simulink model "untitled22"  (R2019a)
settings: Solver=VariableStepAuto  StartTime=0.0  StopTime=100  RelTol=1e-3
values from neighbouring files (symbols this model uses):
  a0 = 3    [Gradient_instant_cost.m]    (also in Gradient_integral_cost.m; MRAC.m = 3+n(1); MRAC2.m = 1+n(1); MRAC3.m = 1)
  a1 = 2    [Gradient_instant_cost.m]    (also in Gradient_integral_cost.m; MRAC.m = 5+n(2); MRAC2.m = 5+n(2); MRAC3.m = 3)
  am = 1    [Untitled34.m]
  b0 = 1    [Gradient_instant_cost.m]    (also in Gradient_integral_cost.m; MRAC.m = 7+n(3); MRAC2.m = 3+n(3); MRAC3.m = 3)
  lambda = [lambda1; lambda0]    [Gradient_instant_cost.m]    (also in Gradient_integral_cost.m; PureLSQ.m; Untitled2.m = 10; Untitled34.m = 1)
settings Model: Creator=Student  LastModifiedBy=Student

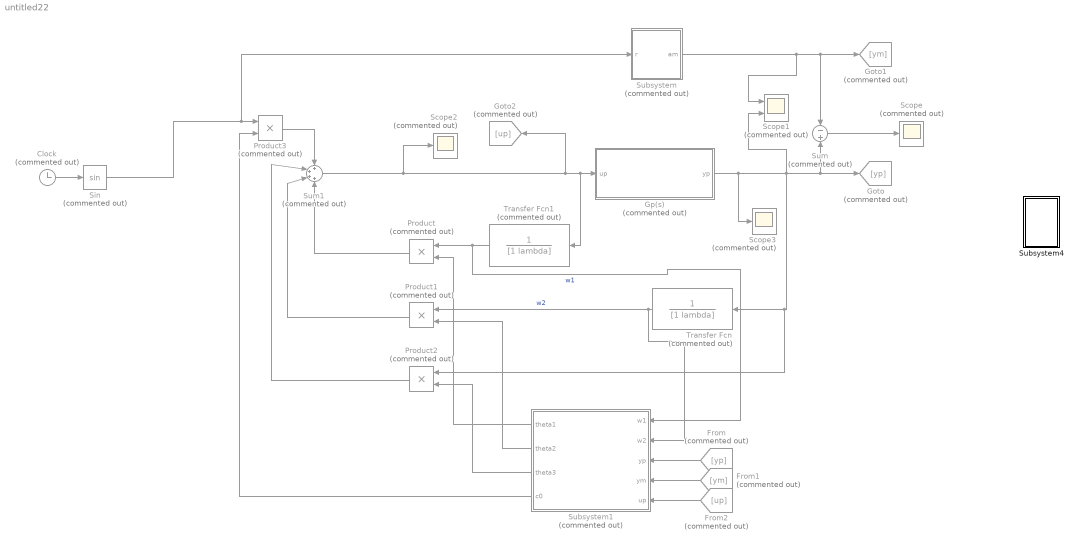
== system untitled22 ==
  Clock : Clock  Commented=on
  From : From  Commented=on  GotoTag=yp
  From1 : From  Commented=on  GotoTag=ym
  From2 : From  Commented=on  GotoTag=up
  Goto : Goto  Commented=on  GotoTag=yp
  Goto1 : Goto  Commented=on  GotoTag=ym
  Goto2 : Goto  Commented=on  GotoTag=up
  Gp(s) : Subsystem  Commented=on
  Product{,1..3} (4 alike) : Product  Commented=on
  Scope : Scope  Commented=on
  Scope1 : Scope  Commented=on  NumInputPorts=2
  Scope2 : Scope  Commented=on
  Scope3 : Scope  Commented=on
  Sin : Trigonometry  Commented=on
  Subsystem : Subsystem  Commented=on
  Subsystem1 : Subsystem  Commented=on
  Subsystem4 : Subsystem
  Sum : Sum  Commented=on  Inputs=-+
  Sum1 : Sum  Commented=on  Inputs=++++
  Transfer Fcn : TransferFcn  Commented=on  Denominator=[1 lambda]
  Transfer Fcn1 : TransferFcn  Commented=on  Denominator=[1 lambda]
  wires:
  Subsystem/1(am) -> Scope1/1, Goto1/1, Sum/1
  Transfer Fcn1/1 -> Subsystem1/1(w1), Product/1  "w1"
  Subsystem1/1(theta1) -> Product/2
  Subsystem1/2(theta2) -> Product1/2
  Transfer Fcn/1 -> Product1/1, Subsystem1/2(w2)  "w2"
  Subsystem1/3(theta3) -> Product2/2
  Product/1 -> Sum1/4
  Product1/1 -> Sum1/3
  Product2/1 -> Sum1/2
  Product3/1 -> Sum1/1
  Subsystem1/4(c0) -> Product3/2
  Gp(s)/1(yp) -> Scope3/1, Product2/1, Transfer Fcn/1, Scope1/2, Goto/1, Sum/2
  From/1 -> Subsystem1/3(yp)
  From1/1 -> Subsystem1/4(ym)
  From2/1 -> Subsystem1/5(up)
  Sum/1 -> Scope/1
  Sin/1 -> Subsystem/1(r), Product3/1
  Sum1/1 -> Scope2/1, Transfer Fcn1/1, Gp(s)/1(up), Goto2/1
  Clock/1 -> Sin/1

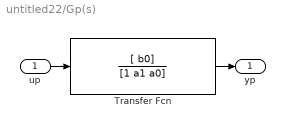
== system untitled22/Gp(s) ==
  up : Inport
  Transfer Fcn : TransferFcn  Numerator=[ b0]  Denominator=[1 a1 a0]
  yp : Outport
  wires:
  Transfer Fcn/1 -> yp/1
  up/1 -> Transfer Fcn/1

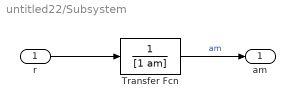
== system untitled22/Subsystem ==
  r : Inport
  Transfer Fcn : TransferFcn  Denominator=[1 am]
  am : Outport
  wires:
  r/1 -> Transfer Fcn/1
  Transfer Fcn/1 -> am/1  "am"

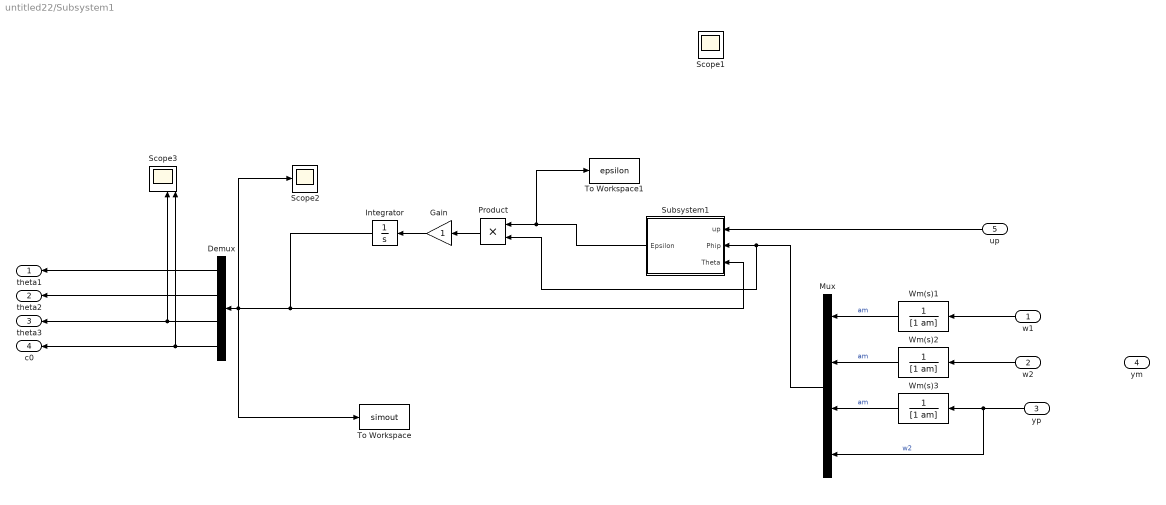
== system untitled22/Subsystem1 ==
  w1 : Inport
  w2 : Inport  Port=2
  yp : Inport  Port=3
  ym : Inport  Port=4
  up : Inport  Port=5
  Demux : Demux
  Gain : Gain
  Integrator : Integrator  InitialCondition=[0;0;0;1]
  Mux : Mux
  Product : Product
  Scope1 : Scope
  Scope2 : Scope
  Scope3 : Scope  NumInputPorts=4
  Subsystem1 : Subsystem
  To Workspace : ToWorkspace  VariableName=simout  SaveFormat=Timeseries  SampleTime=-1
  To Workspace1 : ToWorkspace  VariableName=epsilon  SaveFormat=Timeseries  SampleTime=-1
  Wm(s)1 : TransferFcn  Denominator=[1 am]
  Wm(s)2 : TransferFcn  Denominator=[1 am]
  Wm(s)3 : TransferFcn  Denominator=[1 am]
  theta1 : Outport
  theta2 : Outport  Port=2
  theta3 : Outport  Port=3
  c0 : Outport  Port=4
  wires:
  Demux/3 -> Scope3/3, theta3/1
  Demux/2 -> theta2/1
  Demux/4 -> Scope3/4, c0/1
  Wm(s)1/1 -> Mux/1  "am"
  Wm(s)2/1 -> Mux/2  "am"
  Wm(s)3/1 -> Mux/3  "am"
  Gain/1 -> Integrator/1
  yp/1 -> Mux/4, Wm(s)3/1  "w2"
  Product/1 -> Gain/1
  w1/1 -> Wm(s)1/1
  w2/1 -> Wm(s)2/1
  Demux/1 -> theta1/1
  up/1 -> Subsystem1/1(up)
  Mux/1 -> Product/2, Subsystem1/2(Phip)
  Integrator/1 -> To Workspace/1, Scope2/1, Demux/1, Subsystem1/3(Theta)
  Subsystem1/1("Epsilon ") -> To Workspace1/1, Product/1

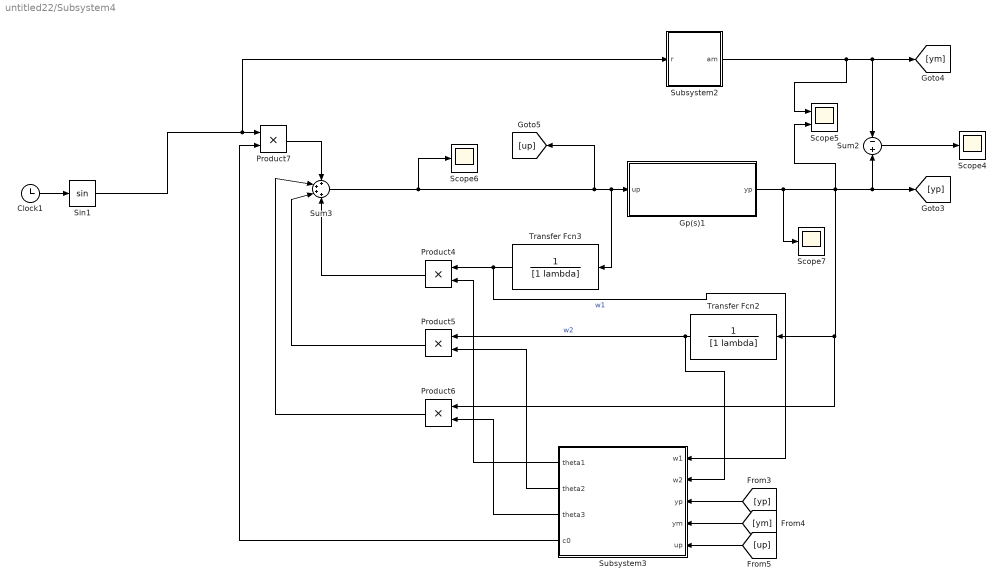
== system untitled22/Subsystem4 ==
  Clock1 : Clock
  Gp(s)1 : Subsystem
  Product{4..7} (4 alike) : Product
  Scope4 : Scope
  Scope5 : Scope  NumInputPorts=2
  Scope6 : Scope
  Scope7 : Scope
  Sin1 : Trigonometry
  Subsystem2 : Subsystem
  Subsystem3 : Subsystem
  Sum2 : Sum  Inputs=-+
  Sum3 : Sum  Inputs=++++
  Transfer Fcn2 : TransferFcn  Denominator=[1 lambda]
  Transfer Fcn3 : TransferFcn  Denominator=[1 lambda]
  wires:
  Gp(s)1/1(yp) -> Scope7/1, Product6/1, Transfer Fcn2/1, Scope5/2, [yp], Sum2/2
  Subsystem3/1(theta1) -> Product4/2
  [ym] -> Subsystem3/4(ym)
  Sum3/1 -> Scope6/1, Transfer Fcn3/1, Gp(s)1/1(up), [up]
  Sin1/1 -> Subsystem2/1(r), Product7/1
  Subsystem2/1(am) -> Scope5/1, [ym], Sum2/1
  Sum2/1 -> Scope4/1
  Product6/1 -> Sum3/2
  [yp] -> Subsystem3/3(yp)
  Product5/1 -> Sum3/3
  Transfer Fcn2/1 -> Product5/1, Subsystem3/2(w2)  "w2"
  Subsystem3/4(c0) -> Product7/2
  [up] -> Subsystem3/5(up)
  Transfer Fcn3/1 -> Subsystem3/1(w1), Product4/1  "w1"
  Product7/1 -> Sum3/1
  Subsystem3/2(theta2) -> Product5/2
  Clock1/1 -> Sin1/1
  Product4/1 -> Sum3/4
  Subsystem3/3(theta3) -> Product6/2

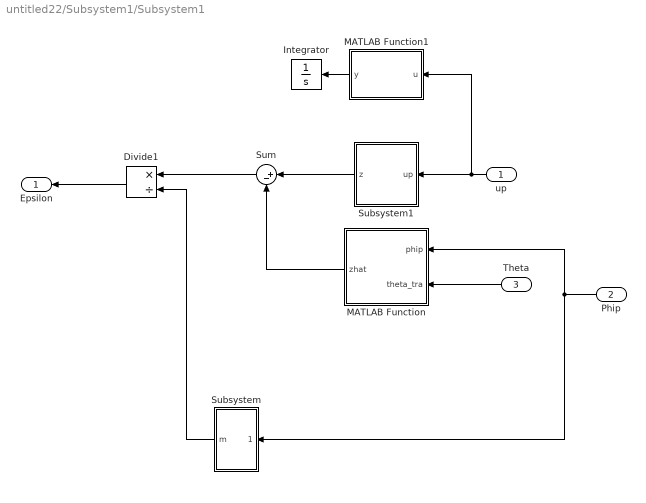
== system untitled22/Subsystem1/Subsystem1 ==
  up : Inport
  Phip : Inport  Port=2
  Theta : Inport  Port=3
  Divide1 : Product  Inputs=*/
  Integrator : Integrator
  MATLAB Function : MATLAB Function  TreatAsAtomicUnit=on
  MATLAB Function1 : MATLAB Function  TreatAsAtomicUnit=on
  Subsystem : Subsystem
  Subsystem1 : Subsystem
  Sum : Sum  Inputs=|+-
  "Epsilon " : Outport
  wires:
  Theta/1 -> MATLAB Function/2(theta_tra)
  Subsystem/1(m) -> Divide1/2
  MATLAB Function/1(zhat) -> Sum/2
  Sum/1 -> Divide1/1
  Phip/1 -> Subsystem/1(phiP), MATLAB Function/1(phip)
  Divide1/1 -> "Epsilon "/1
  up/1 -> MATLAB Function1/1(u), Subsystem1/1(up)
  Subsystem1/1(z) -> Sum/1
  MATLAB Function1/1(y) -> Integrator/1

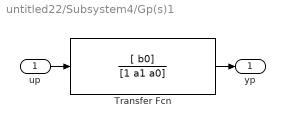
== system untitled22/Subsystem4/Gp(s)1 ==
  up : Inport
  Transfer Fcn : TransferFcn  Numerator=[ b0]  Denominator=[1 a1 a0]
  yp : Outport
  wires:
  Transfer Fcn/1 -> yp/1
  up/1 -> Transfer Fcn/1

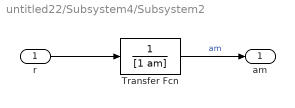
== system untitled22/Subsystem4/Subsystem2 ==
  r : Inport
  Transfer Fcn : TransferFcn  Denominator=[1 am]
  am : Outport
  wires:
  r/1 -> Transfer Fcn/1
  Transfer Fcn/1 -> am/1  "am"

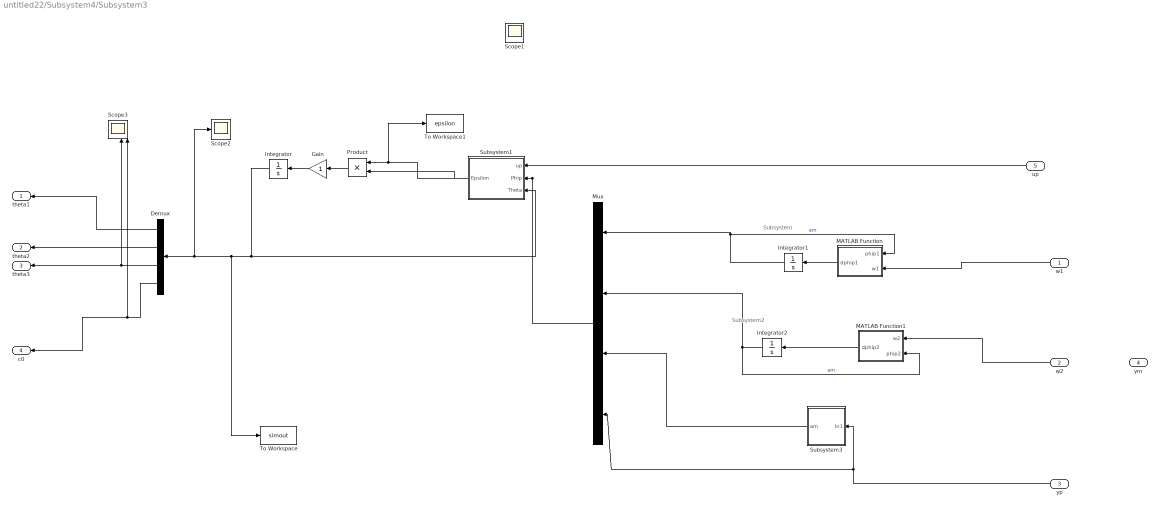
== system untitled22/Subsystem4/Subsystem3 ==
  note: Subsystem2
  note: Subsystem
  w1 : Inport
  w2 : Inport  Port=2
  yp : Inport  Port=3
  ym : Inport  Port=4
  up : Inport  Port=5
  Demux : Demux
  Gain : Gain
  Integrator : Integrator  InitialCondition=[0;0;0;1]
  Integrator1 : Integrator
  Integrator2 : Integrator
  MATLAB Function : MATLAB Function  TreatAsAtomicUnit=on
  MATLAB Function1 : MATLAB Function  TreatAsAtomicUnit=on
  Mux : Mux
  Product : Product
  Scope1 : Scope
  Scope2 : Scope
  Scope3 : Scope  NumInputPorts=4
  Subsystem1 : Subsystem
  Subsystem3 : Subsystem
  To Workspace : ToWorkspace  VariableName=simout  SaveFormat=Timeseries  SampleTime=-1
  To Workspace1 : ToWorkspace  VariableName=epsilon  SaveFormat=Timeseries  SampleTime=-1
  theta1 : Outport
  theta2 : Outport  Port=2
  theta3 : Outport  Port=3
  c0 : Outport  Port=4
  wires:
  Demux/3 -> Scope3/3, theta3/1
  Demux/2 -> theta2/1
  Demux/4 -> Scope3/4, c0/1
  Gain/1 -> Integrator/1
  yp/1 -> Subsystem3/1(In1), Mux/4
  Product/1 -> Gain/1
  Demux/1 -> theta1/1
  up/1 -> Subsystem1/1(up)
  Mux/1 -> Product/2, Subsystem1/2(Phip)
  Integrator/1 -> Demux/1, Scope2/1, To Workspace/1, Subsystem1/3(Theta)
  Subsystem1/1("Epsilon ") -> To Workspace1/1, Product/1
  Subsystem3/1(am) -> Mux/3
  MATLAB Function/1(dphip1) -> Integrator1/1
  Integrator1/1 -> Mux/1, MATLAB Function/1(phip1)  "am"
  w1/1 -> MATLAB Function/2(w1)
  w2/1 -> MATLAB Function1/1(w2)
  MATLAB Function1/1(dphip2) -> Integrator2/1
  Integrator2/1 -> MATLAB Function1/2(phip2), Mux/2  "am"

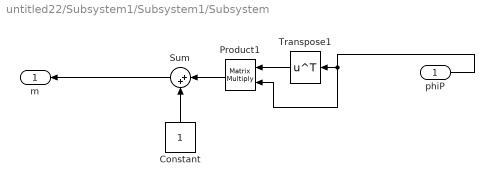
== system untitled22/Subsystem1/Subsystem1/Subsystem ==
  phiP : Inport
  Constant : Constant
  Product1 : Product  Multiplication=Matrix(*)
  Sum : Sum  Inputs=|++
  Transpose1 : Math  Operator=transpose  SaturateOnIntegerOverflow=on
  m : Outport
  wires:
  Product1/1 -> Sum/1
  phiP/1 -> Product1/2, Transpose1/1
  Constant/1 -> Sum/2
  Transpose1/1 -> Product1/1
  Sum/1 -> m/1

== system untitled22/Subsystem1/Subsystem1/Subsystem1 ==
  up : Inport
  Wm(s)4 : TransferFcn  Denominator=[1 am]
  z : Outport
  wires:
  up/1 -> Wm(s)4/1
  Wm(s)4/1 -> z/1  "am"

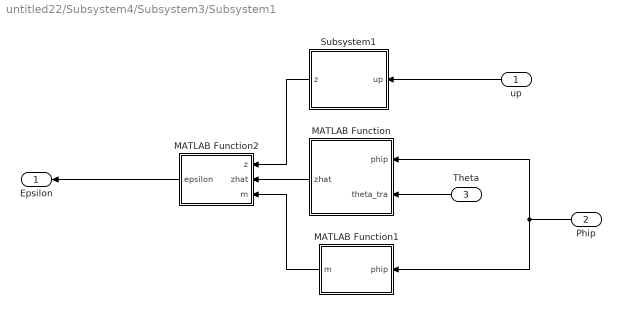
== system untitled22/Subsystem4/Subsystem3/Subsystem1 ==
  up : Inport
  Phip : Inport  Port=2
  Theta : Inport  Port=3
  MATLAB Function : MATLAB Function  TreatAsAtomicUnit=on
  MATLAB Function1 : MATLAB Function  TreatAsAtomicUnit=on
  MATLAB Function2 : MATLAB Function  TreatAsAtomicUnit=on
  Subsystem1 : Subsystem
  "Epsilon " : Outport
  wires:
  Theta/1 -> MATLAB Function/2(theta_tra)
  up/1 -> Subsystem1/1(up)
  Phip/1 -> MATLAB Function/1(phip), MATLAB Function1/1(phip)
  Subsystem1/1(z) -> MATLAB Function2/1(z)
  MATLAB Function/1(zhat) -> MATLAB Function2/2(zhat)
  MATLAB Function1/1(m) -> MATLAB Function2/3(m)
  MATLAB Function2/1(epsilon) -> "Epsilon "/1

== system untitled22/Subsystem4/Subsystem3/Subsystem3 ==
  In1 : Inport
  MATLAB Function : MATLAB Function  TreatAsAtomicUnit=on
  am : Outport
  wires:
  In1/1 -> MATLAB Function/1(phip3)
  MATLAB Function/1(dphip3) -> am/1

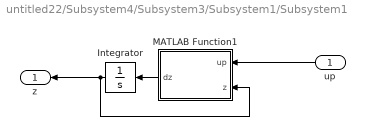
== system untitled22/Subsystem4/Subsystem3/Subsystem1/Subsystem1 ==
  up : Inport
  Integrator : Integrator
  MATLAB Function1 : MATLAB Function  TreatAsAtomicUnit=on
  z : Outport
  wires:
  MATLAB Function1/1(dz) -> Integrator/1
  Integrator/1 -> z/1, MATLAB Function1/2(z)
  up/1 -> MATLAB Function1/1(up)

== matlab function untitled22/Subsystem1/Subsystem1/MATLAB Function1 ==
  data: u input; y output
function y = fcn(u)

y = u;

== matlab function untitled22/Subsystem1/Subsystem1/MATLAB Function ==
  data: phip input; zhat output; theta_tra input
function zhat = fcn(phip, theta_tra)
    zhat = theta_tra'*phip;

== matlab function untitled22/Subsystem4/Subsystem3/Subsystem1/MATLAB Function ==
  data: phip input; zhat output; theta_tra input
function zhat = fcn(phip, theta_tra)
    zhat = theta_tra'*phip;

== matlab function untitled22/Subsystem4/Subsystem3/Subsystem1/Subsystem1/MATLAB Function1 ==
  data: up input; dz output; z input
function dz = fcn(up,z)
    am = 1;
    dz = -am*z + up;

== matlab function untitled22/Subsystem4/Subsystem3/Subsystem1/MATLAB Function1 ==
  data: phip input; m output
function m = fcn(phip)
    m = 1 + phip'*phip;

== matlab function untitled22/Subsystem4/Subsystem3/Subsystem1/MATLAB Function2 ==
  data: z input; epsilon output; zhat input; m input
function epsilon = fcn(z,zhat,m)
    epsilon = (z-zhat)/m;

== matlab function untitled22/Subsystem4/Subsystem3/MATLAB Function ==
  data: phip1 input; dphip1 output; w1 input
function dphip1 = fcn(phip1,w1)
    am  = 1;
    dphip1  = -am*phip1   + w1;

== matlab function untitled22/Subsystem4/Subsystem3/MATLAB Function1 ==
  data: w2 input; dphip2 output; phip2 input
function dphip2 = fcn(w2,phip2)
	am = 1;
    dphip2  = -am*phip2  + w2;

== matlab function untitled22/Subsystem4/Subsystem3/Subsystem3/MATLAB Function ==
  data: phip3 input; dphip3 output; yp input
function dphip3 = fcn(phip3,yp)
    am = 1;
    dphip3  = -am*phip3   + yp;
